simulink model "template_rotativo"  (Simulink 7.2)
settings: Solver=ode1  StartTime=0.0  StopTime=inf  FixedStep=0.002  RelTol=1e-3
PostLoadFcn:
  | qc_set_target_type(getConfigSet(bdroot, 'QUARC Default Target Configuration'));
undefined symbols (not defined in the file or in its folder): HIL
libraries: quarc_library x3, simulink x2, simulink_extras x1
settings Model: Creator=pmartin  LastModifiedBy=aluno  SimulationMode=external  ExtModeTrigDuration=5000
settings SolverCC: PositivePriorityOrder=on
settings OptimizationCC: InitFltsAndDblsToZero=on
settings DebuggingCC: SaveWithParameterizedLinksMsg=none  MultiTaskDSMMsg=warning  MultiTaskCondExecSysMsg=none  StrictBusMsg=None
settings RTWCC: SystemTargetFile=quarc_windows.tlc  TemplateMakefile=quarc_default_tmf  Description=QUARC Win32 Target  ProcessScript=quarc_windows_make_rtw_hook
settings STFCustomTargetCC: TargetPreCompLibLocation=C:\DOCUME~1\ALLUSE~1\DADOSD~1\QUARC\lib\2008b\windows\release  SystemTargetFile=quarc_windows.tlc
settings GRTTargetCC: TargetPreCompLibLocation=C:\DOCUME~1\ALLUSE~1\DADOSD~1\QUARC\lib\2008b\windows\release  CompOptLevelCompliant=off  MatFileLogging=off  ExtMode=on  ExtModeMexFile=quarc_comm

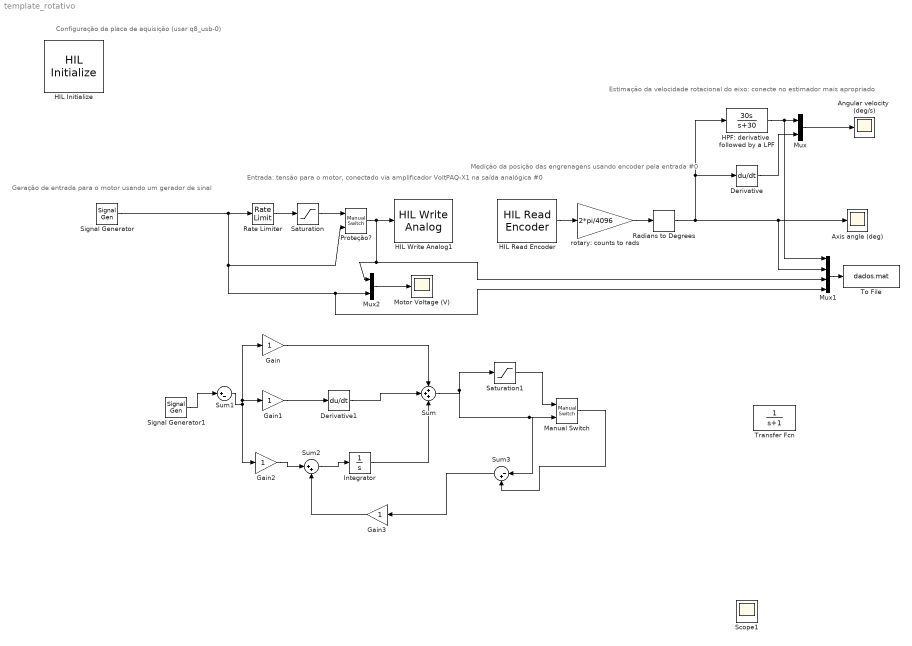
== system template_rotativo ==
  note: Medição da posição das engrenagens usando
      | encoder pela entrada #0
  note: Configuração da placa de aquisição (usar q8_usb-0)
  note: Entrada: tensão para o motor, conectado via
      | amplificador VoltPAQ-X1 na saída analógica #0
  note: Geração de entrada para o motor
      | usando um gerador de sinal
  note: Estimação da velocidade rotacional do eixo:
      | conecte no estimador mais apropriado
  Angular velocity  (deg/s) : Scope
      settings: TickLabels=on  TimeRange=10  YMin=-350  YMax=350  SaveName=data_xc1  DataFormat=Array
  Axis angle (deg) : Scope
      settings: TimeRange=5  YMin=-80  YMax=50
  Derivative : Derivative
  Derivative1 : Derivative
  Gain : Gain  ParameterDataType=sfix(16)  ParameterScaling=2^0  OutDataType=sfix(16)  OutScaling=2^0
  Gain1 : Gain  ParameterDataType=sfix(16)  ParameterScaling=2^0  OutDataType=sfix(16)  OutScaling=2^0
  Gain2 : Gain  ParameterDataType=sfix(16)  ParameterScaling=2^0  OutDataType=sfix(16)  OutScaling=2^0
  Gain3 : Gain  Orientation=left  ParameterDataType=sfix(16)  ParameterScaling=2^0  OutDataType=sfix(16)  OutScaling=2^0
  HIL Initialize : quarc_library/Data Acquisition/Generic/Configuration/HIL Initialize  object_name=HIL-1  board_type=q8_usb  board_number=0  board_options=update_rate=normal  exclusive=off  active=off  hardware_clocks=[0:2]  clock_modes=[]  set_clock_params_at_start=off  set_clock_params_at_switch_in=off  analog_input_channels=[0:7]  analog_input_maximums=10  analog_input_minimums=-10  set_analog_input_params_at_start=on  set_analog_input_params_at_switch_in=off  analog_output_channels=[0:7]  analog_output_maximums=10  analog_output_minimums=-10  initial_analog_outputs=[0]  final_analog_outputs=[0]  watchdog_analog_outputs=0  set_analog_output_params_at_start=on  set_analog_output_params_at_switch_in=off  set_analog_outputs_at_start=on  set_analog_outputs_at_switch_in=off  set_analog_outputs_at_terminate=on  set_analog_outputs_at_switch_out=off  set_analog_outputs_on_watchdog=off  digital_input_channels=[]  digital_output_channels=[0:7]  digital_output_configuration=[]  initial_digital_outputs=[0]  final_digital_outputs=[0]  watchdog_digital_outputs=[0]  set_digital_output_params_at_start=off  set_digital_output_params_at_switch_in=off  set_digital_outputs_at_start=on  set_digital_outputs_at_switch_in=off  set_digital_outputs_at_terminate=on  set_digital_outputs_at_switch_out=off  set_digital_outputs_on_watchdog=off  encoder_channels=[0:7]  quadrature=[4]  encoder_filter_frequency=[]  initial_encoder_counts=[0]  set_encoder_params_at_start=on  set_encoder_params_at_switch_in=off  set_encoder_counts_at_start=on  set_encoder_counts_at_switch_in=off  pwm_channels=[0:7]  pwm_modes=0  pwm_frequency=99.532799999999995e6/4095  pwm_configuration=[0]  pwm_alignment=[0]  pwm_polarity=[1]  pwm_leading_deadband=[0]  pwm_trailing_deadband=[0]  initial_pwm_outputs=[0]  final_pwm_outputs=[0]  watchdog_pwm_outputs=[0]  set_pwm_params_at_start=on  set_pwm_params_at_switch_in=off  set_pwm_outputs_at_start=on  set_pwm_outputs_at_switch_in=off  set_pwm_outputs_at_terminate=on  set_pwm_outputs_at_switch_out=off  set_pwm_outputs_on_watchdog=off  other_output_channels=[]  initial_other_outputs=[]  final_other_outputs=[]  watchdog_other_outputs=[]  set_other_outputs_at_start=off  set_other_outputs_at_switch_in=off  set_other_outputs_at_terminate=off  set_other_outputs_at_switch_out=off  set_other_outputs_on_watchdog=off
  HIL Read Encoder : quarc_library/Data Acquisition/Generic/Immediate I//O/HIL Read Encoder  object_name=HIL-1  channels=[0]  sample_time=qc_get_step_size  active=on  vector_output=off  data_type_mode=Inherit via back propagation  data_type=double
  HIL Write Analog1 : quarc_library/Data Acquisition/Generic/Immediate I//O/HIL Write Analog  object_name=HIL-1  channels=0  sample_time=-1  active=off  vector_input=off
  HPF: derivative  followed by a LPF : TransferFcn  Numerator=[30 0]  Denominator=[1 30]
  Integrator : Integrator
  Manual Switch : simulink/Signal Routing/Manual Switch  SystemSampleTime=-1  sw=1  action=0  varsize=off
  Motor Voltage (V) : Scope
      settings: YMin=-8  YMax=8  SaveName=ScopeData2
  Mux : Mux  Inputs=2
  Mux1 : Mux
  Mux2 : Mux  Inputs=2
  Proteção? : simulink/Signal Routing/Manual Switch  SystemSampleTime=-1  sw=1  action=0  varsize=off
  Radians to Degrees : simulink_extras/Transformations/Radians to Degrees  SystemSampleTime=-1
  Rate Limiter : RateLimiter  RisingSlewLimit=100  FallingSlewLimit=-100  SampleTimeMode=inherited
  Saturation : Saturate  UpperLimit=10  LowerLimit=-10  OutDataType=sfix(16)  OutScaling=2^0
  Saturation1 : Saturate  UpperLimit=10  LowerLimit=-10  OutDataType=sfix(16)  OutScaling=2^0
  Scope1 : Scope
  Signal Generator : SignalGenerator  WaveForm=square  Amplitude=8  Frequency=0.5
  Signal Generator1 : SignalGenerator
  Sum : Sum  Inputs=+++  OutDataType=sfix(16)  OutScaling=2^0
  Sum1 : Sum  Inputs=|+-  OutDataType=sfix(16)  OutScaling=2^0
  Sum2 : Sum  Inputs=|++  OutDataType=sfix(16)  OutScaling=2^0
  Sum3 : Sum  Orientation=left  Inputs=|-+  OutDataType=sfix(16)  OutScaling=2^0
  To File : ToFile  Filename=dados.mat  MatrixName=dados
  Transfer Fcn : TransferFcn  Denominator=[1 1]
  rotary: counts to rads : Gain  Gain=2*pi/4096  SaturateOnIntegerOverflow=on  OutDataTypeStr=Inherit: Same as input  ParamDataTypeStr=Inherit: Same as input
  wires:
  HIL Read Encoder/1 -> rotary: counts to rads/1
  rotary: counts to rads/1 -> Radians to Degrees/1
  HPF: derivative  followed by a LPF/1 -> Mux/1, Mux1/1
  Derivative/1 -> Mux/2
  Mux/1 -> Angular velocity  (deg/s)/1
  Radians to Degrees/1 -> HPF: derivative  followed by a LPF/1, Derivative/1, Axis angle (deg)/1, Mux1/2
  Mux1/1 -> To File/1
  Saturation/1 -> Proteção?/1
  Proteção?/1 -> HIL Write Analog1/1, Mux1/3, Mux2/1
  Rate Limiter/1 -> Saturation/1
  Mux2/1 -> Motor Voltage (V)/1
  Signal Generator/1 -> Rate Limiter/1, Mux2/2, Mux1/4, Proteção?/2
  Derivative1/1 -> Sum/2
  Gain/1 -> Sum/1
  Integrator/1 -> Sum/3
  Gain1/1 -> Derivative1/1
  Signal Generator1/1 -> Sum1/1
  Sum1/1 -> Gain2/1, Gain1/1, Gain/1
  Sum/1 -> Saturation1/1, Manual Switch/2, Sum3/1
  Saturation1/1 -> Manual Switch/1
  Gain2/1 -> Sum2/1
  Sum2/1 -> Integrator/1
  Gain3/1 -> Sum2/2
  Manual Switch/1 -> Sum3/2
  Sum3/1 -> Gain3/1
